simulink model "model"  (R2019b)
settings: Solver=FixedStepDiscrete  StartTime=0.0  StopTime=inf  RelTol=1e-3
undefined symbols (not defined in the file): pause
libraries: simulink x1, dspvision x1, visionsources x1, visionanalysis x1
settings Model: Creator=fabote  LastModifiedBy=fabote

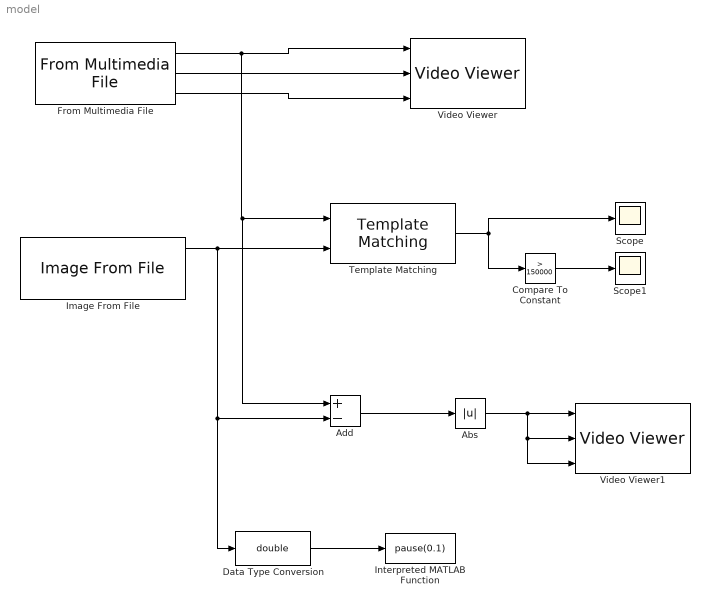
== system model ==
  Abs : Abs
  Add : Sum  Inputs=+-
  Compare To Constant : simulink/Logic and Bit Operations/Compare To Constant  relop=>  const=150000  OutDataTypeStr=boolean
  Data Type Conversion : DataTypeConversion  OutDataTypeStr=double
  From Multimedia File : dspvision/From Multimedia File  inputFilename=/home/fabote/interfejsy/lab3/S2/motion1.avi  readRange=[1 Inf]  loop=on  numPlays=inf  outputStreams=Video only  videoDataType=uint8  audioDataType=int16  inheritSampleTime=on  userDefinedSampleTime=1/30  noAudioOutput=off  isIntensityVideo=off  fourcc=RGB  colorVideoFormat=Separate color signals  outputEOF=off  dataOrg=Column-major  audioFrameSize=1024  computeAudioFrameSize=off  outSamplingMode=Sample based
      settings: SourceProductName=DSP System Toolbox  SourceProductBaseCode=DS
  Image From File : visionsources/Image From File  Tag=vipblks_nd  FileName=/home/fabote/interfejsy/lab3/S2/tlo0000.bmp  Ts=inf  imagePorts=Separate color signals  OutPortLabels=R|G|B  ImageDataType=Inherit from input image  sdImageDataType=uint(8)  Signed=on  WordLength=16  FractionLengthMode=User-defined  FractionLength=15
      settings: SourceProductName=Computer Vision Toolbox
  Interpreted MATLAB Function : MATLABFcn  MATLABFcn=pause(0.1)  OutputDimensions=0
  Scope : Scope
  Scope1 : Scope
  Template Matching : visionanalysis/Template Matching  metric=Sum of absolute differences  output=Metric matrix  method=Exhaustive  nMetric=off  nSize=3  roi=off  roiValid=off  roundingMode=Floor  overflowMode=off  prodOutputMode=Binary point scaling  prodOutputWordLength=32  prodOutputFracLength=0  prodOutputSlope=2^0  accumMode=Binary point scaling  accumWordLength=32  accumFracLength=0  accumSlope=2^0  outputMode=Binary point scaling  outputWordLength=32  outputFracLength=0  outputSlope=2^0
      settings: SourceProductName=Computer Vision Toolbox  SourceProductBaseCode=VP
  Video Viewer : VideoViewer  imagePorts=separate color signals  FigPos=[47 713 408 311]
  Video Viewer1 : VideoViewer  imagePorts=separate color signals  FigPos=[1329 705 428 297]
  wires:
  From Multimedia File/1 -> Add/1, Template Matching/1, Video Viewer/1
  From Multimedia File/2 -> Video Viewer/2
  From Multimedia File/3 -> Video Viewer/3
  Image From File/1 -> Add/2, Data Type Conversion/1, Template Matching/2
  Template Matching/1 -> Scope/1, Compare To Constant/1
  Compare To Constant/1 -> Scope1/1
  Data Type Conversion/1 -> Interpreted MATLAB Function/1
  Abs/1 -> Video Viewer1/3, Video Viewer1/2, Video Viewer1/1
  Add/1 -> Abs/1
